simulink model "TBRe_Mod"  (R2017b)
settings: Solver=FixedStepDiscrete  StartTime=0.0  StopTime=inf  FixedStep=0.0001  RelTol=1e-3
PostLoadFcn:
  | model_init();
values from neighbouring files (symbols this model uses):
  SOC_Calc_bPoint = Simulink.Parameter    [ecuparams.m]
  SOC_Calc_Data = Simulink.Parameter    [ecuparams.m]
  Voltage_Act_bPoint = Simulink.Parameter    [ecuparams.m]
  Voltage_Act_Data = Simulink.Parameter    [ecuparams.m]
undefined symbols (not defined in the file or in its folder): _240Nm_Breakpoint, _240Nm_Data, Brake_Active_Threshold, Brk1_OOR_High, Brk1_OOR_Low, Brk2_OOR_High, Brk2_OOR_Low, Motor_To_Road_Speed_Ratio, Throttle_Active_Threshold, Throttle_Torque_Map_
libraries: simulink x26
(part 8 of 8)

== stateflow chart TBRe_Mod/MainTask/Vehicle_Functionality_Layer/Vehicle_Operation_Mode/TS Enable ==
  note: Start here
  state Default_State
    entry:
    TS_Enable = 0;
    State = 0;
    Reset_Out = 0;
  state Precharge
    entry:
    TS_Enable = 1;
    State = 1;
    Reset_Out =1;
  state HV_System_Deactivating
    entry:
    TS_Enable = 0;
    State = 3;
    Reset_Out = 0;
  state HV_System_Active
    entry:
    TS_Enable = 1;
    State = 2;
    Reset_Out = 0;
  (default) -> Default_State
  HV_System_Deactivating -> Default_State [order 1] : after(0.5,sec)
  Precharge -> Default_State [order 3] : [after(0.5,sec)]
  (junction 86) -> Default_State
  Default_State -> Precharge : [hasChangedFrom(btnPreCharge, 0) && btnPreCharge && after(1,sec)]
  Precharge -> (junction 86) [order 2] : [Shutdown]
  HV_System_Deactivating -> (junction 86) [order 2] : [Shutdown]
  HV_System_Active -> (junction 86) [order 1] : [Shutdown || ~LowAIR_Status]
  (junction 95) -> (junction 86) [order 2] : [Shutdown || ~LowAIR_Status]
  HV_System_Active -> HV_System_Deactivating [order 2] : [hasChangedFrom(btnPreCharge, 0) && btnPreCharge && after(0.5,sec)]
  Precharge -> (junction 95) [order 1] : [LowAIR_Status]
  (junction 95) -> HV_System_Active [order 1] : [after(0.5,sec)]
  data: btnPreCharge input boolean; LowAIR_Status input boolean; Shutdown input boolean; TS_Enable output boolean; State output uint8; Reset_Out output boolean; Latch_Status input boolean
